simulink subsystem "Sensors"  (R2024b)
settings: Solver=VariableStepAuto  StartTime=0.0  StopTime=10.0  RelTol=1e-3
undefined symbols (not defined in the file): SimIn
libraries: simulink x1
settings Model: Creator=macheson  LastModifiedBy=macheson

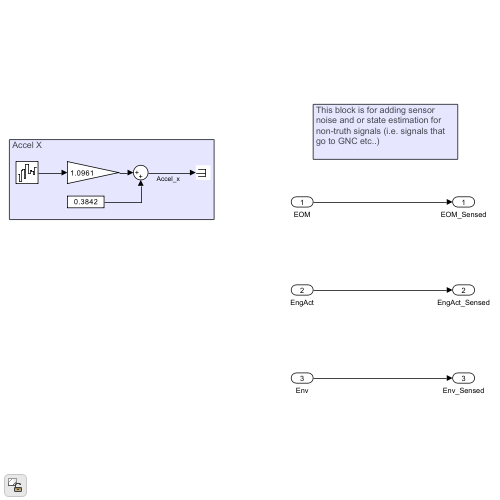
[thumbnail: Simulink's stored preview of the top-level diagram]
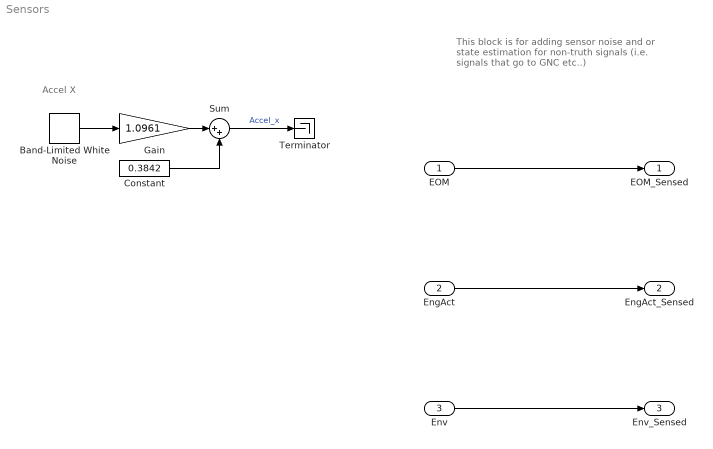
== system Sensors ==
  note: Accel X
  note: This block is for adding sensor
      | noise and or state estimation for
      | non-truth signals (i.e. signals that
      | go to GNC etc..)
  EOM : Inport
  EngAct : Inport  Port=2
  Env : Inport  Port=3
  Band-Limited White Noise : simulink/Sources/Band-Limited White Noise  Cov=1  Ts=SimIn.model_params.sim_rate  seed=[23341]
  Constant : Constant  Value=0.3842
  Gain : Gain  Gain=1.0961
  Sum : Sum  Inputs=|++
  Terminator : Terminator
  EOM_Sensed : Outport
  EngAct_Sensed : Outport  Port=2
  Env_Sensed : Outport  Port=3
  wires:
  Env/1 -> Env_Sensed/1
  EngAct/1 -> EngAct_Sensed/1
  EOM/1 -> EOM_Sensed/1
  Band-Limited White Noise/1 -> Gain/1
  Gain/1 -> Sum/1
  Constant/1 -> Sum/2
  Sum/1 -> Terminator/1  "Accel_x"
